simulink model "OutputToVisualizationTrialByTrial"  (R2016b)
settings: Solver=FixedStepDiscrete  StartTime=0.0  StopTime=10.0  FixedStep=sCoreParams.core.stepPeriod  RelTol=1e-3  EnableMultiTasking=on
undefined symbols (not defined in the file): sCoreParams, sCoreParams_viz_featureInds
libraries: slrtlib x2, xpcrtudplib x2, dspsigops x1, xpcutilitieslib x1, xpcobsoletelib x1
settings Model: DataTypeOverride=Double  MinMaxOverflowLogging=ForceOff  Creator=rzelmann  LastModifiedBy=Rack_Deux
settings SolverCC: EnableConcurrentExecution=on  ConcurrentTasks=on  AutoInsertRateTranBlk=on
settings DataIOCC: SaveFormat=StructureWithTime  SaveOutput=off  SignalLogging=off  DSMLogging=off  SaveTime=off
settings OptimizationCC: BlockReduction=off  DefaultParameterBehavior=Inlined  LifeSpan=inf
settings DebuggingCC: AllowSymbolicDim=off  SFUnexpectedBacktrackingDiag=warning  SFNoUnconditionalDefaultTransitionDiag=warning  SFExecutionAtInitializationDiag=none
settings HardwareCC: ProdBitPerPointer=32  ProdBitPerSizeT=32  ProdBitPerPtrDiffT=32  ProdLargestAtomicFloat=None  ProdWordSize=32  ProdLongLongMode=on  ProdHWDeviceType=Generic->32-bit x86 compatible
settings ModelReferenceCC: UpdateModelReferenceTargets=Force  ParallelModelReferenceMATLABWorkerInit=Load Top Model  ModelReferenceNumInstancesAllowed=Single  ModelReferencePassRootInputsByReference=off
settings RTWCC: SystemTargetFile=slrt.tlc  TemplateMakefile=slrt_default_tmf  Description=Simulink Real-Time  RTWCompilerOptimization=on
settings CodeAppCC: MaxIdLength=63
settings ConfigComp: CovMetricSettings=dw  CovHtmlReporting=on  CovSaveCumulativeToWorkspaceVar=on  CovSaveSingleToWorkspaceVar=on  CovExternalEMLEnable=off

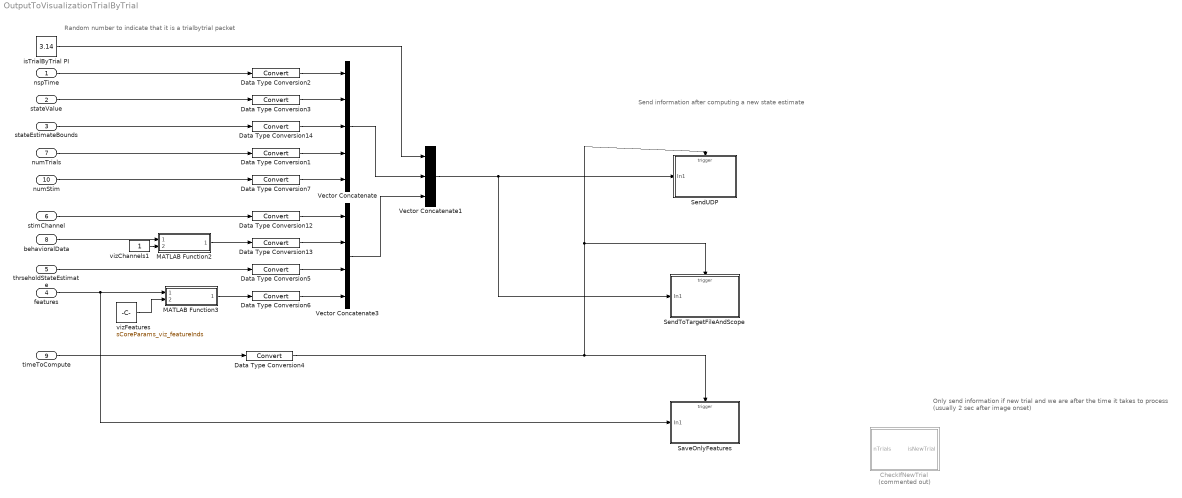
== system OutputToVisualizationTrialByTrial ==
  note: Random number to indicate that it is a trialbytrial packet
  note: Send information after computing a new state estimate
  note: Only send information if new trial
      | and we are after the time it takes to process (usually 2 sec after image onset)
  nspTime : Inport  SampleTime=sCoreParams.core.stepPeriod
  stateValue : Inport  Port=2  OutDataTypeStr=double  SampleTime=sCoreParams.core.stepPeriod
  stateEstimateBounds : Inport  Port=3  OutDataTypeStr=double  PortDimensions=[1 2]  SampleTime=sCoreParams.core.stepPeriod
  features : Inport  Port=4  PortDimensions=[sCoreParams.decoders.txDetector.nDataPointsUsedInDetection sCoreParams.decoders.txDetector.nFeaturesUsedInDetection]  SampleTime=sCoreParams.core.stepPeriod
  thrseholdStateEstimate : Inport  Port=5  PortDimensions=2  SampleTime=sCoreParams.core.stepPeriod
  stimChannel : Inport  Port=6  OutDataTypeStr=int32  PortDimensions=[1 2]  SampleTime=sCoreParams.core.stepPeriod  Interpolate=off
  numTrials : Inport  Port=7  SampleTime=sCoreParams.core.stepPeriod
  behavioralData : Inport  Port=8  PortDimensions=[sCoreParams.core.samplesPerStep 1]  SampleTime=sCoreParams.core.stepPeriod  Interpolate=off
  timeToCompute : Inport  Port=9  OutDataTypeStr=boolean  PortDimensions=1  SampleTime=sCoreParams.core.stepPeriod
  numStim : Inport  Port=10  SampleTime=sCoreParams.core.stepPeriod
  CheckIfNewTrial : Subsystem  Commented=on
  Data Type Conversion{1..7,12..14} (10 alike) : DataTypeConversion
  MATLAB Function2 : MATLAB Function  TreatAsAtomicUnit=on
  MATLAB Function3 : MATLAB Function  TreatAsAtomicUnit=on
  SaveOnlyFeatures : Subsystem
  SendToTargetFileAndScope : Subsystem
  SendUDP : Subsystem
  Vector Concatenate : Concatenate  NumInputs=5
  Vector Concatenate1 : Concatenate  NumInputs=3
  Vector Concatenate3 : Concatenate  NumInputs=4
  isTrialByTrial PI : Constant  Value=3.14
  vizChannels1 : Constant
  vizFeatures : Constant  Value=sCoreParams_viz_featureInds
  wires:
  features/1 -> SaveOnlyFeatures/1(In1), MATLAB Function3/1(signalIn)
  Data Type Conversion2/1 -> Vector Concatenate/1
  MATLAB Function3/1(signalOut) -> Data Type Conversion6/1
  Vector Concatenate/1 -> Vector Concatenate1/2
  Vector Concatenate3/1 -> Vector Concatenate1/3
  Vector Concatenate1/1 -> SendToTargetFileAndScope/1(In1), SendUDP/1(In1)
  vizFeatures/1 -> MATLAB Function3/2(selectCh)
  stimChannel/1 -> Data Type Conversion12/1
  nspTime/1 -> Data Type Conversion2/1
  stateValue/1 -> Data Type Conversion3/1
  thrseholdStateEstimate/1 -> Data Type Conversion5/1
  numTrials/1 -> Data Type Conversion1/1
  Data Type Conversion13/1 -> Vector Concatenate3/2
  Data Type Conversion5/1 -> Vector Concatenate3/3
  MATLAB Function2/1(signalOut) -> Data Type Conversion13/1
  behavioralData/1 -> MATLAB Function2/1(signalIn)
  vizChannels1/1 -> MATLAB Function2/2(selectCh)
  stateEstimateBounds/1 -> Data Type Conversion14/1
  Data Type Conversion14/1 -> Vector Concatenate/3
  timeToCompute/1 -> Data Type Conversion4/1
  Data Type Conversion3/1 -> Vector Concatenate/2
  Data Type Conversion1/1 -> Vector Concatenate/4
  Data Type Conversion12/1 -> Vector Concatenate3/1
  isTrialByTrial PI/1 -> Vector Concatenate1/1
  Data Type Conversion4/1 -> SaveOnlyFeatures/Trigger, SendToTargetFileAndScope/Trigger, SendUDP/Trigger
  Data Type Conversion6/1 -> Vector Concatenate3/4
  numStim/1 -> Data Type Conversion7/1
  Data Type Conversion7/1 -> Vector Concatenate/5

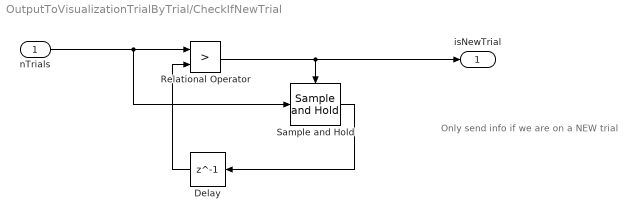
== system OutputToVisualizationTrialByTrial/CheckIfNewTrial ==
  note: Only send info if we are on a NEW trial
  nTrials : Inport
  Delay : Delay  DelayLength=1
  Relational Operator : RelationalOperator  Operator=>  OutDataTypeStr=boolean  RndMeth=Simplest
  Sample and Hold : dspsigops/Sample and Hold  trig=Rising edge  initCond=0  latchinput=off
  isNewTrial : Outport
  wires:
  Delay/1 -> Relational Operator/2
  Sample and Hold/1 -> Delay/1
  Relational Operator/1 -> Sample and Hold/Trigger, isNewTrial/1
  nTrials/1 -> Sample and Hold/1, Relational Operator/1

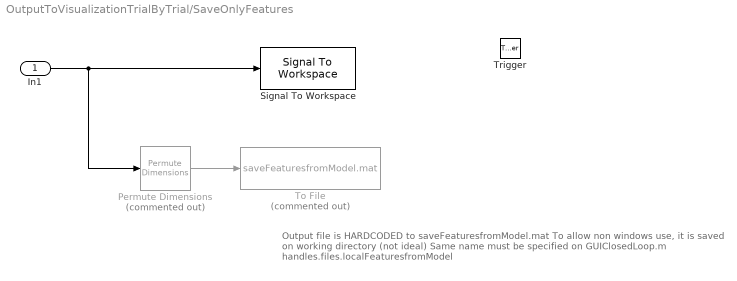
== system OutputToVisualizationTrialByTrial/SaveOnlyFeatures ==
  note: Output file is HARDCODED to saveFeaturesfromModel.mat
      | To allow non windows use, it is saved on working directory (not ideal)
      | Same name must be specified on GUIClosedLoop.m handles.files.localFeaturesfromModel
  In1 : Inport
  Trigger : TriggerPort  VariantControl=Variant  PortDimensions=1
  Permute Dimensions : PermuteDimensions  Commented=on
  Signal To Workspace : SignalToWorkspace  VariableName=savedFeatures
      settings: CopyFcn=dspblkcopystw(gcbh);
  "To File " : ToFile  Commented=on  Filename=saveFeaturesfromModel.mat  MatrixName=savedFeaturesfromModel  SaveFormat=Timeseries
  wires:
  In1/1 -> Permute Dimensions/1, Signal To Workspace/1
  Permute Dimensions/1 -> "To File "/1

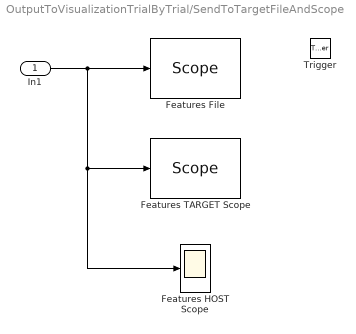
== system OutputToVisualizationTrialByTrial/SendToTargetFileAndScope ==
  In1 : Inport
  Trigger : TriggerPort  VariantControl=Variant  PortDimensions=1
  Features File : slrtlib/Displays and Logging/Scope   scopeno=2  scopetype=File  autostart=on  viewmode=Graphical redraw  formatstr='%15.6f'  grid=on  ylimits=[0,0]  nosamples=1000  noprepostsamples=-10  interleave=1  triggermode=FreeRun  triggersignal=1  trigsignalfromport=on  triggerlevel=0.0  triggerslope=Rising  triggerscope=1  triggersample=0  filename=feat_<%%%>.dat  mode=Lazy  writesize=512  autorestart=on  dynamicfilemode=on  maxwritefilesize=512*1024^2
  Features HOST Scope : Scope
  Features TARGET Scope : slrtlib/Displays and Logging/Scope   scopeno=3  scopetype=Target  autostart=on  viewmode=Graphical sliding  formatstr='%15.6f'  grid=on  ylimits=[0,0]  nosamples=1000  noprepostsamples=0  interleave=1  triggermode=FreeRun  triggersignal=1  trigsignalfromport=on  triggerlevel=0.0  triggerslope=Rising  triggerscope=1  triggersample=0  filename=data.dat  mode=Lazy  writesize=512  autorestart=off  dynamicfilemode=off  maxwritefilesize=512*1024^2
  wires:
  In1/1 -> Features HOST Scope/1, Features TARGET Scope/1, Features File/1

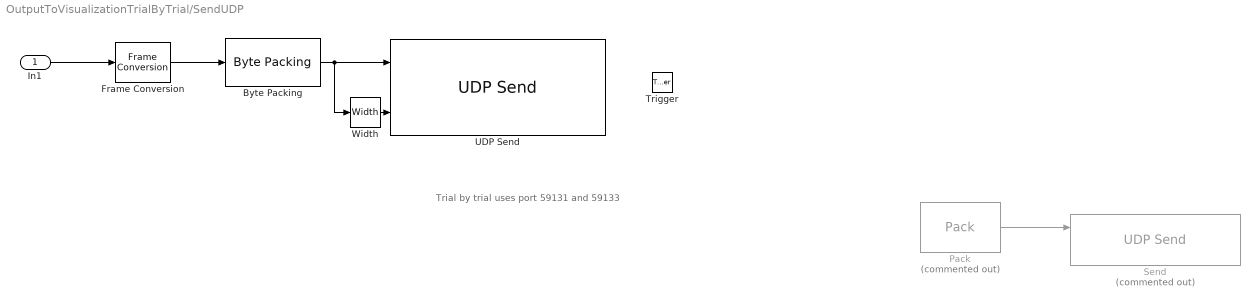
== system OutputToVisualizationTrialByTrial/SendUDP ==
  note: Trial by trial uses port 59131 and 59133
  In1 : Inport
  Trigger : TriggerPort  VariantControl=Variant  PortDimensions=1
  "Byte Packing " : xpcutilitieslib/Byte Packing   MaskPackedDataType=uint8  MaskUnpackedDataTypes={'double'}  MaskAlignment=1
  Frame Conversion : FrameConversion  InheritSamplingMode=off  OutFrame=Sample-based
  Pack : xpcobsoletelib/Utilities/Pack   Commented=on  datatypes={'double'}  byteAlign=1
  Send : xpcrtudplib/UDP Send  Commented=on  ipAddressVal=Use host-target connection  localPort=59121  toAddress=255.255.255.255  toPort=59123  sampleTime=-1
  UDP Send : xpcrtudplib/UDP Send  ipAddressVal=Use host-target connection  localPort=59131  toAddress=255.255.255.255  toPort=59133  sampleTime=-1
  Width : Width
  wires:
  "Byte Packing "/1 -> Width/1, UDP Send/1
  In1/1 -> Frame Conversion/1
  Frame Conversion/1 -> "Byte Packing "/1
  Pack/1 -> Send/1
  Width/1 -> UDP Send/2

== matlab function OutputToVisualizationTrialByTrial/MATLAB Function2 ==
  data: signalIn input; signalOut output size=[1 1]; selectCh input
function signalOut = selectChannelsFromFrame(signalIn,selectCh)
%#codegen
signalOut = signalIn(end,selectCh); %Only send first time point of frame
%signalOut = selectChannelsFromFrame_EML(signalIn,selectCh);

== matlab function OutputToVisualizationTrialByTrial/MATLAB Function3 ==
  data: signalIn input; signalOut output size=[1 length(sCoreParams_viz_featureInds)]; selectCh input
function signalOut = selectChannels(signalIn,selectCh)
%#codegen
%signalOut = signalIn(:,selectCh);
signalOut = signalIn(end,selectCh);
%signalOut = selectChannels_EML(signalIn,selectCh);
